simulink model "AnalysisSimAP_2016a"  (R2016a)
settings: Solver=VariableStepAuto  StartTime=0.0  StopTime=80  RelTol=1e-3
values from neighbouring files (symbols this model uses):
  Csim_discrete = c2d(Csim,1/151,'tustin')    [RobustnessAnalysisAP.m]    (also in RobustnessAnalysis_MIL9490.m)
  GeriFDsysPID2_IO = NdofwActSens(okeep,ikeep,AEC6,ModeShape,FEM,Vmps,aeroProp,massProp,     coeffdataPIDfull,actdata,sensdata)    [GenerateGeriModelAP.m]    (also in RobustnessAnalysisAP.m = P; RobustnessAnalysis_MIL9490.m = P)
  RFS = min([RFS_ICM_P, RFS_ICM_G, RFS_OCM_P, RFS_OCM_G])    [CalculateRobustFlutterSpeed.m]    (also in RobustnessAnalysisAP.m = min([RFSIPM,RFSIGM,RFSOPM,RFSOGM]); RobustnessAnalysis_MIL9490.m = min([RFSIPM,RFSIGM,RFSOPM,RFSOGM]))
  RLfall = -30    [RobustnessAnalysisAP.m]    (also in RobustnessAnalysis_MIL9490.m)
  RLrise = 30    [RobustnessAnalysisAP.m]    (also in RobustnessAnalysis_MIL9490.m)
  Sathi = 30    [RobustnessAnalysisAP.m]    (also in RobustnessAnalysis_MIL9490.m)
  Satlw = -30    [RobustnessAnalysisAP.m]    (also in RobustnessAnalysis_MIL9490.m)
  Vinf = Vinfs    [RobustnessAnalysisAP.m]    (also in RobustnessAnalysis_MIL9490.m; example_geri.mat = [25 26 27 28 29 30 31 32 33 34 35 36 ... (21 elements, 1x21))
undefined symbols (not defined in the file or in its folder): K
libraries: simulink_extras x7, cstblocks x5
settings Model: Creator=Julian  LastModifiedBy=juliant
settings GRTTargetCC: GeneratePreprocessorConditionals=Use local settings

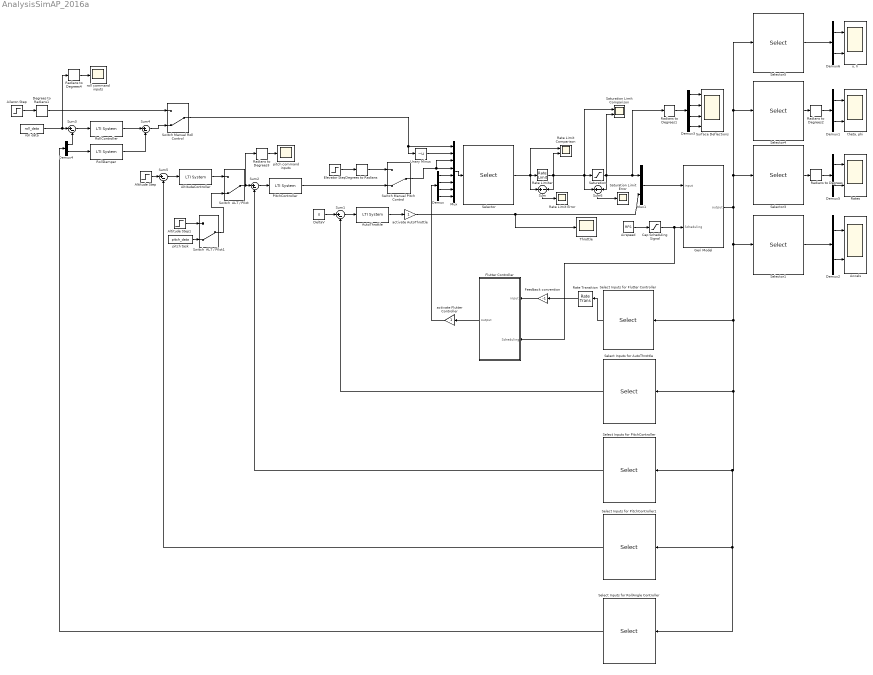
== system AnalysisSimAP_2016a ==
  Accels : Scope  NumInputPorts=2
  Aileron Step : Step  Time=3  After=0  SampleTime=0
  Airspeed : Constant  Value=RFS
  Altitude Step : Step  After=25  SampleTime=0
  Altitude Step1 : Step  After=15/180*pi  SampleTime=0
  AltitudeController : cstblocks/LTI System  sys=AltitudeController  IC=[]
  AutoThrottle : cstblocks/LTI System  sys=AutoThrottle  IC=[]
  Cap Scheduling Signal : Saturate  UpperLimit=45  LowerLimit=25
  Degrees to Radians : simulink_extras/Transformations/Degrees to Radians
  Degrees to Radians1 : simulink_extras/Transformations/Degrees to Radians
  DeltaV : Constant  Value=0
  Demux : Demux  Outputs=[1 1 1 1]
  Demux{1,4..6} (4 alike) : Demux  Outputs=2
  Demux2 : Demux  Outputs=[3 3]
  Demux3 : Demux  Outputs=[2 2 2 2]
  Elevator Step : Step  SampleTime=0
  Feedback convention : Gain  Gain=-1
  Flutter Controller : Subsystem
  Geri Model : Subsystem
  Mux : Mux  Inputs=8
  Mux1 : Mux  Inputs=[8 1]
  PitchController : cstblocks/LTI System  sys=PitchController  IC=[]
  Radians to Degrees{,1..4} (5 alike) : simulink_extras/Transformations/Radians to Degrees
  Rate Limit Comparison : Scope  NumInputPorts=2
  Rate Limit Error : Scope
  Rate Limiter : RateLimiter  RisingSlewLimit=RLrise/180*pi  FallingSlewLimit=RLfall/180*pi  SampleTimeMode=inherited
  Rate Transition : RateTransition  OutPortSampleTime=1/151
  Rates : Scope  NumInputPorts=2
  RollController : cstblocks/LTI System  sys=RollController  IC=[]
  RollDamper : cstblocks/LTI System  sys=RollDamper  IC=[]
  Saturation : Saturate  UpperLimit=Sathi/180*pi  LowerLimit=Satlw/180*pi
  Saturation Limit Error : Scope
  Saturation Limit Comparison : Scope  NumInputPorts=2
  Select Inputs for AutoThrottle : Selector  InputPortWidth=12  IndexOptions=Index vector (dialog)  Indices=1  OutputSizes=1
  Select Inputs for Flutter Controller : Selector  InputPortWidth=12  IndexOptions=Index vector (dialog)  Indices=5:12  OutputSizes=1
  Select Inputs for PitchController : Selector  InputPortWidth=12  IndexOptions=Index vector (dialog)  Indices=2  OutputSizes=1
  Select Inputs for PitchController1 : Selector  InputPortWidth=12  IndexOptions=Index vector (dialog)  Indices=3  OutputSizes=1
  Select Inputs for RollAngle Controller : Selector  InputPortWidth=12  IndexOptions=Index vector (dialog)  Indices=[4 6]  OutputSizes=1
  Selector : Selector  InputPortWidth=8  IndexOptions=Index vector (dialog)  Indices=[5 6 1 2 3 4 7 8]  OutputSizes=1
  Selector1 : Selector  InputPortWidth=12  IndexOptions=Index vector (dialog)  Indices=[12 8 11 10 7 9]  OutputSizes=1
  Selector3 : Selector  InputPortWidth=12  IndexOptions=Index vector (dialog)  Indices=[5 6]  OutputSizes=1
  Selector4 : Selector  InputPortWidth=12  IndexOptions=Index vector (dialog)  Indices=[2 4]  OutputSizes=1
  Selector5 : Selector  InputPortWidth=12  IndexOptions=Index vector (dialog)  Indices=[1 3]  OutputSizes=1
  Sum : Sum  Inputs=+-
  Sum{1..5} (5 alike) : Sum  Inputs=|+-
  Sum6 : Sum  Inputs=+-
  Surface Deflections : Scope  NumInputPorts=4
  Switch  ALT / Pilot : ManualSwitch  CurrentSetting=0
  Switch  ALT / Pilot1 : ManualSwitch  CurrentSetting=0
  Switch Manual Pitch Control : ManualSwitch  CurrentSetting=0
  Switch Manual Roll Control : ManualSwitch  CurrentSetting=0
  Throttle : Scope
  Unary Minus : UnaryMinus
  activate AutoThrottle : Gain
  activate Flutter Controller : Gain
  pitch command inputs : Scope
  pitch task : FromWorkspace  VariableName=pitch_data  SampleTime=0
  roll command inputs : Scope
  roll data : FromWorkspace  VariableName=roll_data  SampleTime=0
  "theta, phi" : Scope  NumInputPorts=2
  "u, h" : Scope  NumInputPorts=2
  wires:
  Cap Scheduling Signal/1 -> Flutter Controller/2(Scheduling), Geri Model/2(Scheduling)
  Airspeed/1 -> Cap Scheduling Signal/1
  Mux/1 -> Selector/1
  Flutter Controller/1(output) -> activate Flutter Controller/1
  Demux/4 -> Mux/8
  Demux/3 -> Mux/7
  Demux/2 -> Mux/6
  Demux/1 -> Mux/5
  Switch Manual Pitch Control/1 -> Mux/3, Mux/4
  Aileron Step/1 -> Degrees to Radians1/1
  Switch Manual Roll Control/1 -> Mux/1, Unary Minus/1
  Selector3/1 -> Radians to Degrees/1
  Geri Model/1(output) -> Selector5/1, Selector4/1, Selector3/1, Select Inputs for RollAngle Controller/1, Select Inputs for PitchController1/1, Select Inputs for PitchController/1, Select Inputs for AutoThrottle/1, Select Inputs for Flutter Controller/1, Selector1/1
  Selector1/1 -> Demux2/1
  Demux2/1 -> Accels/1
  Demux2/2 -> Accels/2
  Radians to Degrees/1 -> Demux5/1
  Radians to Degrees1/1 -> Demux3/1
  Demux3/1 -> Surface Deflections/1
  Demux3/3 -> Surface Deflections/3
  Demux3/2 -> Surface Deflections/2
  Demux3/4 -> Surface Deflections/4
  Saturation/1 -> Sum6/2, Saturation Limit Comparison/2, Radians to Degrees1/1, Mux1/1
  Rate Limiter/1 -> Sum6/1, Saturation Limit Comparison/1, Saturation/1, Sum/2, Rate Limit Comparison/2
  Sum/1 -> Rate Limit Error/1
  Select Inputs for Flutter Controller/1 -> Rate Transition/1
  AutoThrottle/1 -> activate AutoThrottle/1
  Select Inputs for AutoThrottle/1 -> Sum1/2
  Sum1/1 -> AutoThrottle/1
  DeltaV/1 -> Sum1/1
  Elevator Step/1 -> Degrees to Radians/1
  Sum2/1 -> PitchController/1
  Select Inputs for PitchController/1 -> Sum2/2
  Sum4/1 -> Switch Manual Roll Control/2
  Sum3/1 -> RollController/1
  Select Inputs for RollAngle Controller/1 -> Demux4/1
  PitchController/1 -> Switch Manual Pitch Control/2
  Switch  ALT / Pilot1/1 -> Switch  ALT / Pilot/2
  roll data/1 -> Radians to Degrees4/1, Sum3/1
  RollController/1 -> Sum4/1
  RollDamper/1 -> Sum4/2
  Demux4/2 -> RollDamper/1
  Demux4/1 -> Sum3/2
  Selector/1 -> Sum/1, Rate Limit Comparison/1, Rate Limiter/1
  Radians to Degrees2/1 -> Demux1/1
  Selector4/1 -> Radians to Degrees2/1
  Selector5/1 -> Demux6/1
  Demux1/1 -> "theta, phi"/1
  Demux1/2 -> "theta, phi"/2
  Demux5/1 -> Rates/1
  Demux5/2 -> Rates/2
  Unary Minus/1 -> Mux/2
  activate AutoThrottle/1 -> Throttle/1, Mux1/2
  Mux1/1 -> Geri Model/1(input)
  Select Inputs for PitchController1/1 -> Sum5/2
  Switch  ALT / Pilot/1 -> Radians to Degrees3/1, Sum2/1
  AltitudeController/1 -> Switch  ALT / Pilot/1
  Sum5/1 -> AltitudeController/1
  Altitude Step/1 -> Sum5/1
  Sum6/1 -> Saturation Limit Error/1
  Degrees to Radians1/1 -> Switch Manual Roll Control/1
  Degrees to Radians/1 -> Switch Manual Pitch Control/1
  Rate Transition/1 -> Feedback convention/1
  activate Flutter Controller/1 -> Demux/1
  Demux6/1 -> "u, h"/1
  Demux6/2 -> "u, h"/2
  Radians to Degrees4/1 -> roll command inputs/1
  Radians to Degrees3/1 -> pitch command inputs/1
  Feedback convention/1 -> Flutter Controller/1(input)
  pitch task/1 -> Switch  ALT / Pilot1/2
  Altitude Step1/1 -> Switch  ALT / Pilot1/1

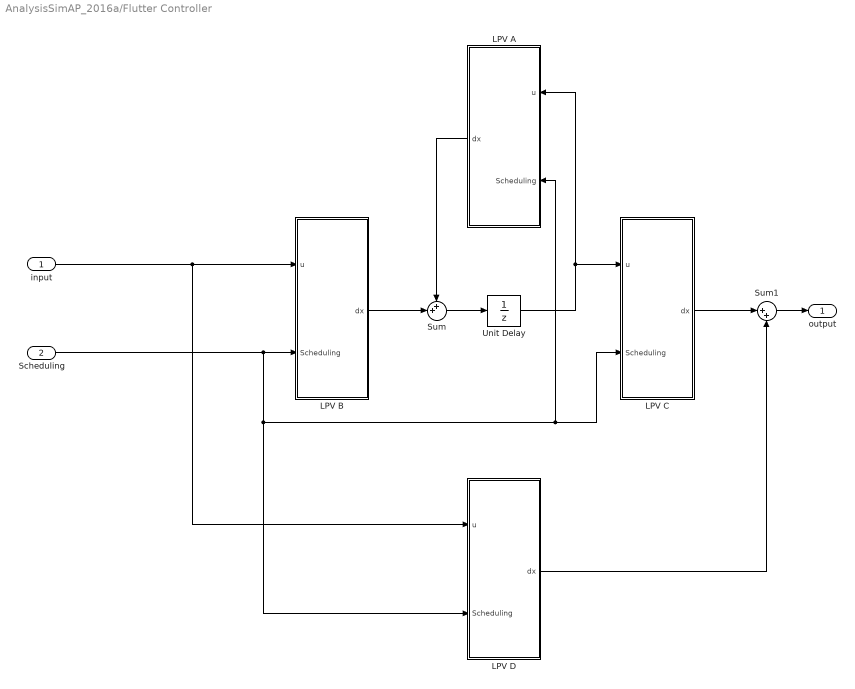
== system AnalysisSimAP_2016a/Flutter Controller ==
  input : Inport
  Scheduling : Inport  Port=2
  LPV A : Subsystem
  LPV B : Subsystem
  LPV C : Subsystem
  LPV D : Subsystem
  Sum : Sum  Inputs=++|
  Sum1 : Sum  Inputs=|++
  Unit Delay : UnitDelay  SampleTime=-1
  output : Outport
  wires:
  LPV C/1(dx) -> Sum1/1
  Sum/1 -> Unit Delay/1
  Unit Delay/1 -> LPV C/1(u), LPV A/1(u)
  input/1 -> LPV D/1(u), LPV B/1(u)
  Scheduling/1 -> LPV B/2(Scheduling), LPV D/2(Scheduling), LPV C/2(Scheduling), LPV A/2(Scheduling)
  LPV B/1(dx) -> Sum/2
  LPV A/1(dx) -> Sum/1
  Sum1/1 -> output/1
  LPV D/1(dx) -> Sum1/2

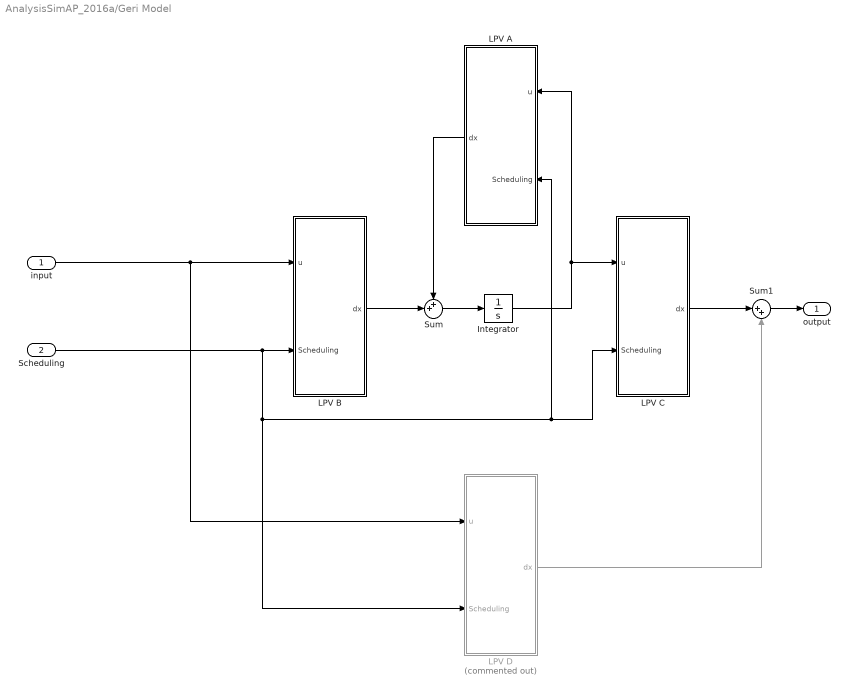
== system AnalysisSimAP_2016a/Geri Model ==
  input : Inport
  Scheduling : Inport  Port=2
  Integrator : Integrator  InitialCondition=zeros(size(GeriFDsysPID2_IO.a,1),1)
  LPV A : Subsystem
  LPV B : Subsystem
  LPV C : Subsystem
  LPV D : Subsystem  Commented=on
  Sum : Sum  Inputs=++|
  Sum1 : Sum  Inputs=|++
  output : Outport
  wires:
  LPV C/1(dx) -> Sum1/1
  Sum/1 -> Integrator/1
  Integrator/1 -> LPV C/1(u), LPV A/1(u)
  input/1 -> LPV D/1(u), LPV B/1(u)
  Scheduling/1 -> LPV B/2(Scheduling), LPV D/2(Scheduling), LPV C/2(Scheduling), LPV A/2(Scheduling)
  LPV B/1(dx) -> Sum/2
  LPV A/1(dx) -> Sum/1
  Sum1/1 -> output/1
  LPV D/1(dx) -> Sum1/2

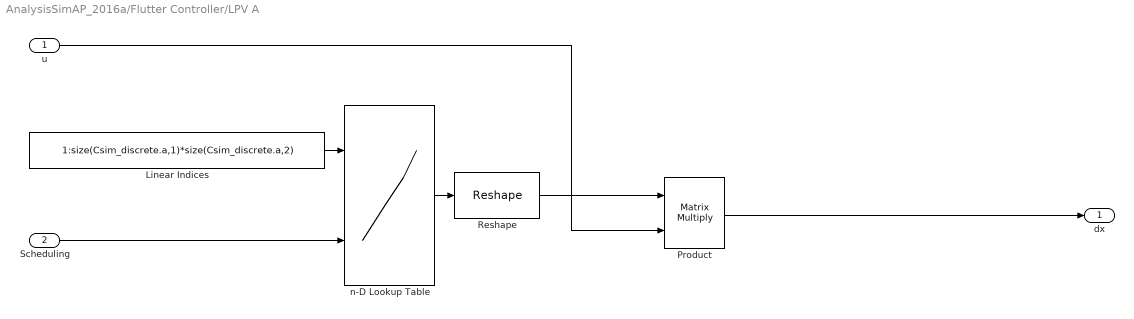
== system AnalysisSimAP_2016a/Flutter Controller/LPV A ==
  u : Inport
  Scheduling : Inport  Port=2
  Linear Indices : Constant  Value=1:size(Csim_discrete.a,1)*size(Csim_discrete.a,2)
  Product : Product  Multiplication=Matrix(*)
  Reshape : Reshape  OutputDimensionality=Customize  OutputDimensions=[size(Csim_discrete.a,1),size(Csim_discrete.a,2)]
  n-D Lookup Table : Lookup_n-D  BreakpointsForDimension1=1:size(Csim_discrete.a,1)*size(Csim_discrete.a,2)  BreakpointsForDimension2=Vinf  BreakpointsForDimension3=K.Parameter.q2.GridData  BreakpointsForDimension4=K.Parameter.q3.GridData  BreakpointsForDimension5=q3.GridData  BeginIndexSearchUsingPreviousIndexResult=on  Table=reshape(Csim_discrete.a,[size(Csim_discrete.a,1)*size(Csim_discrete.a,2), numel(Vinf)])  ExtrapMethod=Clip  UseLastTableValue=on  InternalRulePriority=Speed  RndMeth=Simplest  InputSameDT=on
  dx : Outport
  wires:
  Scheduling/1 -> n-D Lookup Table/2
  u/1 -> Product/2
  Linear Indices/1 -> n-D Lookup Table/1
  Reshape/1 -> Product/1
  n-D Lookup Table/1 -> Reshape/1
  Product/1 -> dx/1

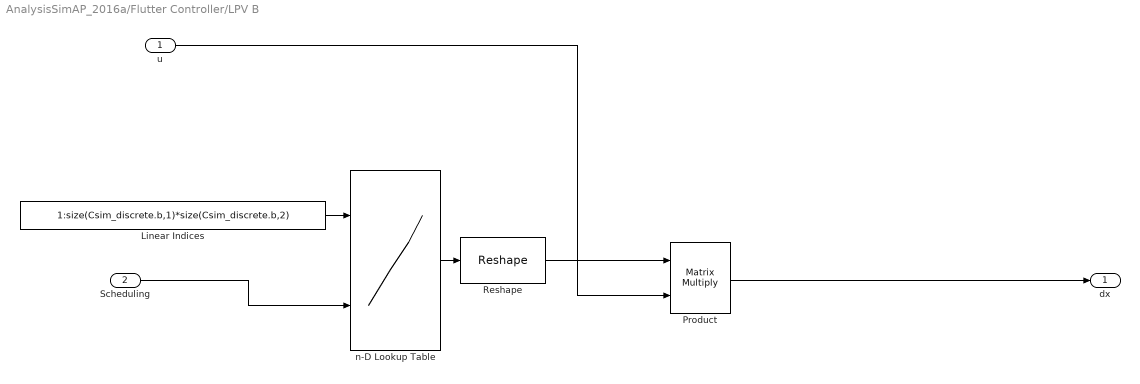
== system AnalysisSimAP_2016a/Flutter Controller/LPV B ==
  u : Inport
  Scheduling : Inport  Port=2
  Linear Indices : Constant  Value=1:size(Csim_discrete.b,1)*size(Csim_discrete.b,2)
  Product : Product  Multiplication=Matrix(*)
  Reshape : Reshape  OutputDimensionality=Customize  OutputDimensions=[size(Csim_discrete.b,1),size(Csim_discrete.b,2)]
  n-D Lookup Table : Lookup_n-D  BreakpointsForDimension1=1:size(Csim_discrete.b,1)*size(Csim_discrete.b,2)  BreakpointsForDimension2=Vinf  BreakpointsForDimension3=K.Parameter.q2.GridData  BreakpointsForDimension4=K.Parameter.q3.GridData  BreakpointsForDimension5=q3.GridData  BeginIndexSearchUsingPreviousIndexResult=on  Table=reshape(Csim_discrete.b,[size(Csim_discrete.b,1)*size(Csim_discrete.b,2), numel(Vinf)])  ExtrapMethod=Clip  UseLastTableValue=on  InternalRulePriority=Speed  RndMeth=Simplest  InputSameDT=on
  dx : Outport
  wires:
  Product/1 -> dx/1
  n-D Lookup Table/1 -> Reshape/1
  Reshape/1 -> Product/1
  Linear Indices/1 -> n-D Lookup Table/1
  u/1 -> Product/2
  Scheduling/1 -> n-D Lookup Table/2

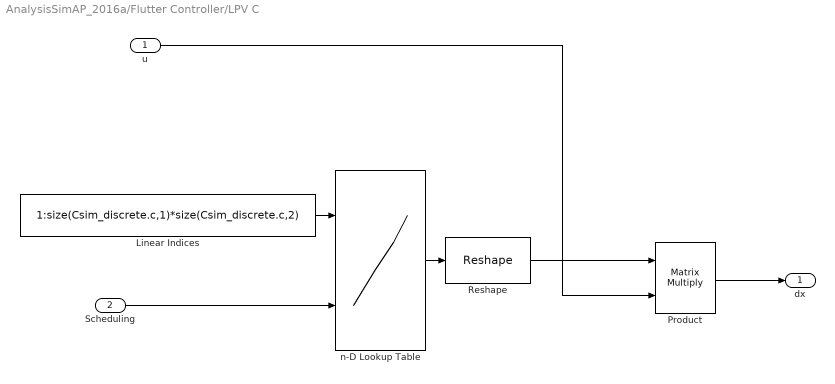
== system AnalysisSimAP_2016a/Flutter Controller/LPV C ==
  u : Inport
  Scheduling : Inport  Port=2
  Linear Indices : Constant  Value=1:size(Csim_discrete.c,1)*size(Csim_discrete.c,2)
  Product : Product  Multiplication=Matrix(*)
  Reshape : Reshape  OutputDimensionality=Customize  OutputDimensions=[size(Csim_discrete.c,1),size(Csim_discrete.c,2)]
  n-D Lookup Table : Lookup_n-D  BreakpointsForDimension1=1:size(Csim_discrete.c,1)*size(Csim_discrete.c,2)  BreakpointsForDimension2=Vinf  BreakpointsForDimension3=K.Parameter.q2.GridData  BreakpointsForDimension4=K.Parameter.q3.GridData  BreakpointsForDimension5=q3.GridData  Table=reshape(Csim_discrete.c,[size(Csim_discrete.c,1)*size(Csim_discrete.c,2), numel(Vinf)])  ExtrapMethod=Clip  UseLastTableValue=on  InternalRulePriority=Speed  RndMeth=Simplest  InputSameDT=on
  dx : Outport
  wires:
  Scheduling/1 -> n-D Lookup Table/2
  u/1 -> Product/2
  Linear Indices/1 -> n-D Lookup Table/1
  Reshape/1 -> Product/1
  n-D Lookup Table/1 -> Reshape/1
  Product/1 -> dx/1

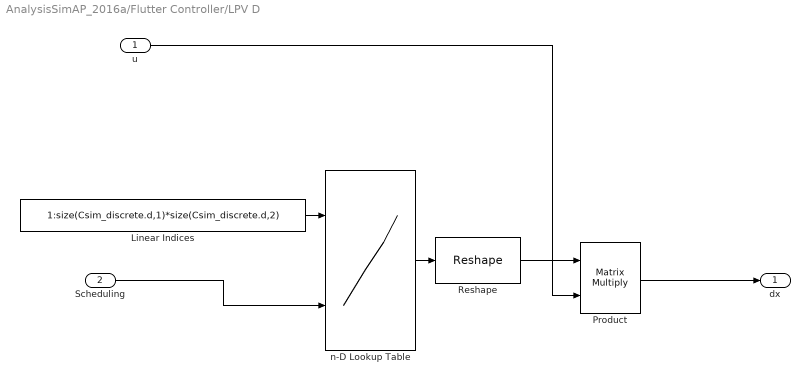
== system AnalysisSimAP_2016a/Flutter Controller/LPV D ==
  u : Inport
  Scheduling : Inport  Port=2
  Linear Indices : Constant  Value=1:size(Csim_discrete.d,1)*size(Csim_discrete.d,2)
  Product : Product  Multiplication=Matrix(*)
  Reshape : Reshape  OutputDimensionality=Customize  OutputDimensions=[size(Csim_discrete.d,1),size(Csim_discrete.d,2)]
  n-D Lookup Table : Lookup_n-D  BreakpointsForDimension1=1:size(Csim_discrete.d,1)*size(Csim_discrete.d,2)  BreakpointsForDimension2=Vinf  BreakpointsForDimension3=K.Parameter.q2.GridData  BreakpointsForDimension4=K.Parameter.q3.GridData  BreakpointsForDimension5=q3.GridData  Table=reshape(Csim_discrete.d,[size(Csim_discrete.d,1)*size(Csim_discrete.d,2), numel(Vinf)])  ExtrapMethod=Clip  UseLastTableValue=on  InternalRulePriority=Speed  RndMeth=Simplest  InputSameDT=on
  dx : Outport
  wires:
  Product/1 -> dx/1
  n-D Lookup Table/1 -> Reshape/1
  Reshape/1 -> Product/1
  Linear Indices/1 -> n-D Lookup Table/1
  u/1 -> Product/2
  Scheduling/1 -> n-D Lookup Table/2

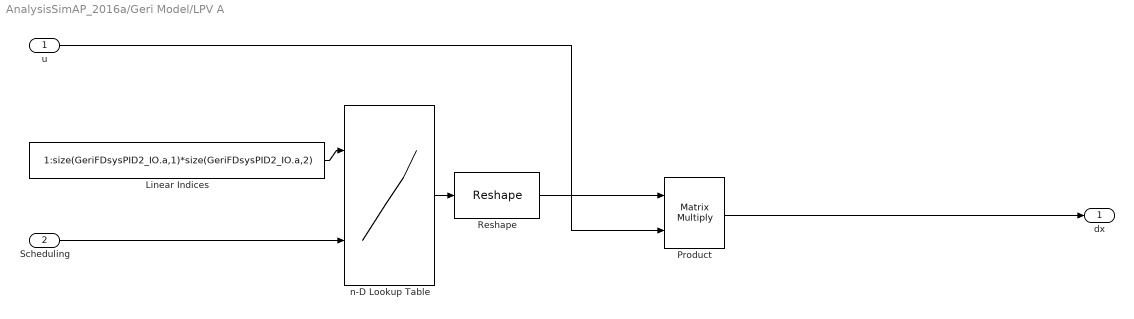
== system AnalysisSimAP_2016a/Geri Model/LPV A ==
  u : Inport
  Scheduling : Inport  Port=2
  Linear Indices : Constant  Value=1:size(GeriFDsysPID2_IO.a,1)*size(GeriFDsysPID2_IO.a,2)
  Product : Product  Multiplication=Matrix(*)
  Reshape : Reshape  OutputDimensionality=Customize  OutputDimensions=[size(GeriFDsysPID2_IO.a,1),size(GeriFDsysPID2_IO.a,2)]
  n-D Lookup Table : Lookup_n-D  BreakpointsForDimension1=1:size(GeriFDsysPID2_IO.a,1)*size(GeriFDsysPID2_IO.a,2)  BreakpointsForDimension2=Vinf  BreakpointsForDimension3=K.Parameter.q2.GridData  BreakpointsForDimension4=K.Parameter.q3.GridData  BreakpointsForDimension5=q3.GridData  BeginIndexSearchUsingPreviousIndexResult=on  Table=reshape(GeriFDsysPID2_IO.a,[size(GeriFDsysPID2_IO.a,1)*size(GeriFDsysPID2_IO.a,2), numel(Vinf)])  ExtrapMethod=Clip  UseLastTableValue=on  InternalRulePriority=Speed  RndMeth=Simplest  InputSameDT=on
  dx : Outport
  wires:
  Scheduling/1 -> n-D Lookup Table/2
  u/1 -> Product/2
  Linear Indices/1 -> n-D Lookup Table/1
  Reshape/1 -> Product/1
  n-D Lookup Table/1 -> Reshape/1
  Product/1 -> dx/1

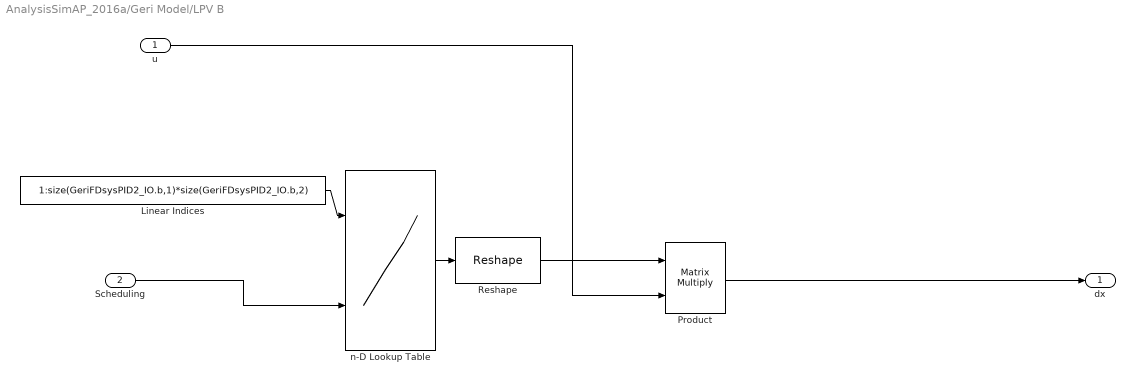
== system AnalysisSimAP_2016a/Geri Model/LPV B ==
  u : Inport
  Scheduling : Inport  Port=2
  Linear Indices : Constant  Value=1:size(GeriFDsysPID2_IO.b,1)*size(GeriFDsysPID2_IO.b,2)
  Product : Product  Multiplication=Matrix(*)
  Reshape : Reshape  OutputDimensionality=Customize  OutputDimensions=[size(GeriFDsysPID2_IO.b,1),size(GeriFDsysPID2_IO.b,2)]
  n-D Lookup Table : Lookup_n-D  BreakpointsForDimension1=1:size(GeriFDsysPID2_IO.b,1)*size(GeriFDsysPID2_IO.b,2)  BreakpointsForDimension2=Vinf  BreakpointsForDimension3=K.Parameter.q2.GridData  BreakpointsForDimension4=K.Parameter.q3.GridData  BreakpointsForDimension5=q3.GridData  BeginIndexSearchUsingPreviousIndexResult=on  Table=reshape(GeriFDsysPID2_IO.b,[size(GeriFDsysPID2_IO.b,1)*size(GeriFDsysPID2_IO.b,2), numel(Vinf)])  ExtrapMethod=Clip  UseLastTableValue=on  InternalRulePriority=Speed  RndMeth=Simplest  InputSameDT=on
  dx : Outport
  wires:
  Product/1 -> dx/1
  n-D Lookup Table/1 -> Reshape/1
  Reshape/1 -> Product/1
  Linear Indices/1 -> n-D Lookup Table/1
  u/1 -> Product/2
  Scheduling/1 -> n-D Lookup Table/2

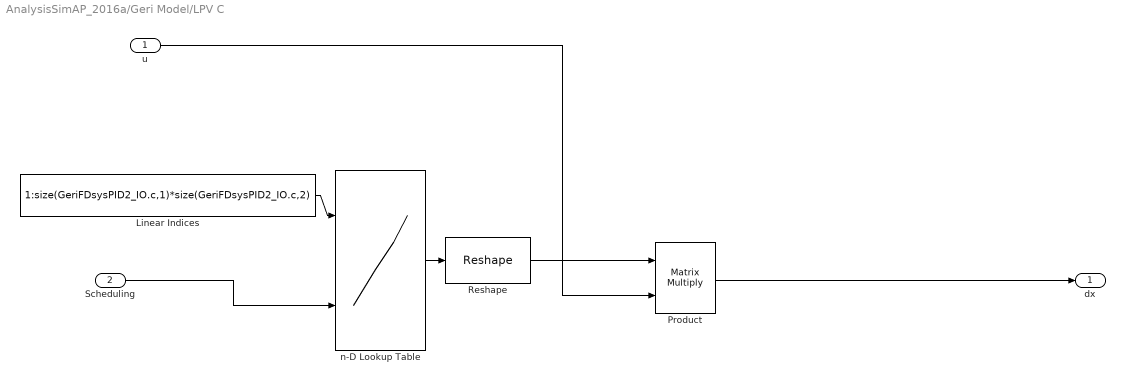
== system AnalysisSimAP_2016a/Geri Model/LPV C ==
  u : Inport
  Scheduling : Inport  Port=2
  Linear Indices : Constant  Value=1:size(GeriFDsysPID2_IO.c,1)*size(GeriFDsysPID2_IO.c,2)
  Product : Product  Multiplication=Matrix(*)
  Reshape : Reshape  OutputDimensionality=Customize  OutputDimensions=[size(GeriFDsysPID2_IO.c,1),size(GeriFDsysPID2_IO.c,2)]
  n-D Lookup Table : Lookup_n-D  BreakpointsForDimension1=1:size(GeriFDsysPID2_IO.c,1)*size(GeriFDsysPID2_IO.c,2)  BreakpointsForDimension2=Vinf  BreakpointsForDimension3=K.Parameter.q2.GridData  BreakpointsForDimension4=K.Parameter.q3.GridData  BreakpointsForDimension5=q3.GridData  Table=reshape(GeriFDsysPID2_IO.c,[size(GeriFDsysPID2_IO.c,1)*size(GeriFDsysPID2_IO.c,2), numel(Vinf)])  ExtrapMethod=Clip  UseLastTableValue=on  InternalRulePriority=Speed  RndMeth=Simplest  InputSameDT=on
  dx : Outport
  wires:
  Scheduling/1 -> n-D Lookup Table/2
  u/1 -> Product/2
  Linear Indices/1 -> n-D Lookup Table/1
  Reshape/1 -> Product/1
  n-D Lookup Table/1 -> Reshape/1
  Product/1 -> dx/1

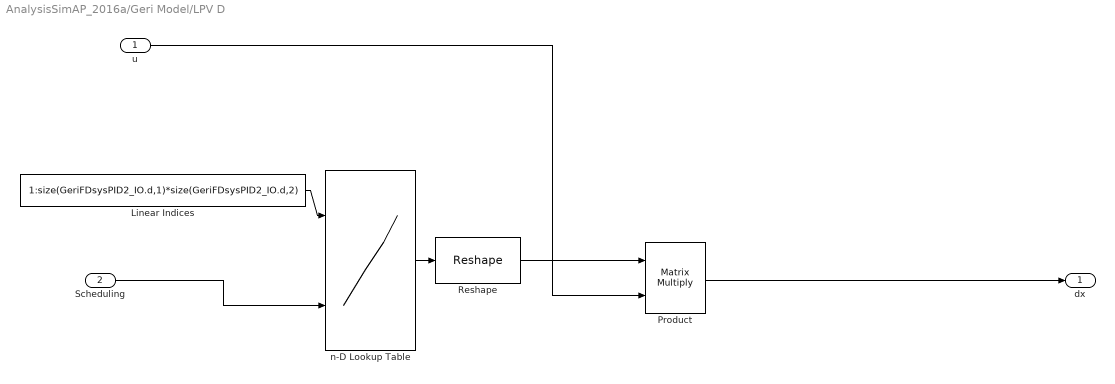
== system AnalysisSimAP_2016a/Geri Model/LPV D ==
  u : Inport
  Scheduling : Inport  Port=2
  Linear Indices : Constant  Value=1:size(GeriFDsysPID2_IO.d,1)*size(GeriFDsysPID2_IO.d,2)
  Product : Product  Multiplication=Matrix(*)
  Reshape : Reshape  OutputDimensionality=Customize  OutputDimensions=[size(GeriFDsysPID2_IO.d,1),size(GeriFDsysPID2_IO.d,2)]
  n-D Lookup Table : Lookup_n-D  BreakpointsForDimension1=1:size(GeriFDsysPID2_IO.d,1)*size(GeriFDsysPID2_IO.d,2)  BreakpointsForDimension2=Vinf  BreakpointsForDimension3=K.Parameter.q2.GridData  BreakpointsForDimension4=K.Parameter.q3.GridData  BreakpointsForDimension5=q3.GridData  Table=reshape(GeriFDsysPID2_IO.d,[size(GeriFDsysPID2_IO.d,1)*size(GeriFDsysPID2_IO.d,2), numel(Vinf)])  ExtrapMethod=Clip  UseLastTableValue=on  InternalRulePriority=Speed  RndMeth=Simplest  InputSameDT=on
  dx : Outport
  wires:
  Product/1 -> dx/1
  n-D Lookup Table/1 -> Reshape/1
  Reshape/1 -> Product/1
  Linear Indices/1 -> n-D Lookup Table/1
  u/1 -> Product/2
  Scheduling/1 -> n-D Lookup Table/2
